simulink model "cosmic_ray_system_top"  (R2019a)
settings: Solver=VariableStepAuto  StartTime=0.0  StopTime=10.0  RelTol=1e-3
libraries: xbsIndex_r4 x3434, casper_library_misc x148, xps_library x3, casper_library_delays x1
(part 9 of 27)

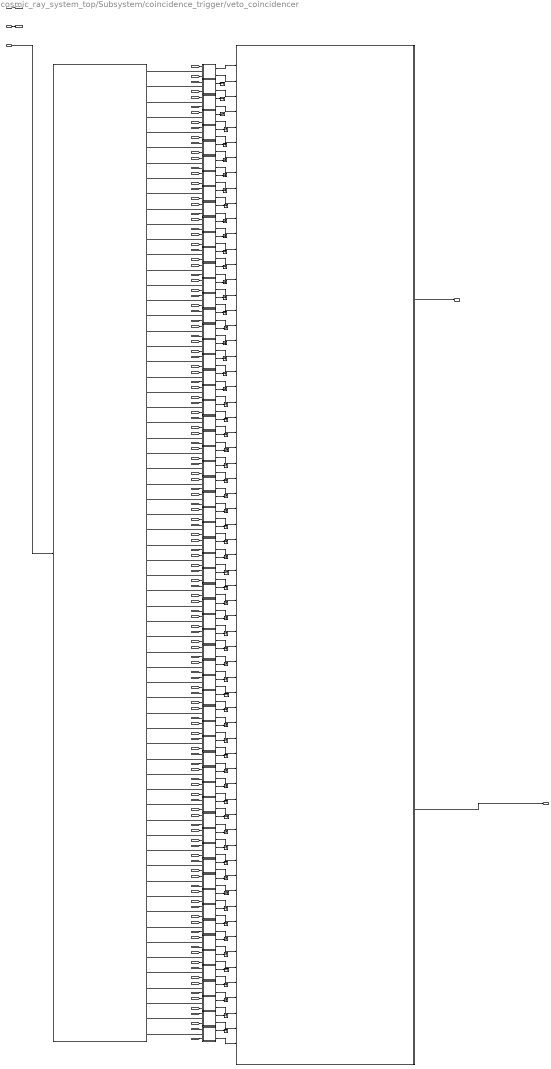
== system cosmic_ray_system_top/Subsystem/coincidence_trigger/veto_coincidencer ==
  window_length : Inport
  data_bus_in : Inport  Port=2
  sync_in : Inport  Port=3
  Terminator{,1..62} (63 alike) : Terminator
  adder_tree : Subsystem  AncestorBlock=casper_library_misc/adder_tree  mask(adder_tree){n_inputs=64, csp_latency=1, adder_imp=Fabric, first_stage_hdl=on, floating_point=off, dvalid_en=off, float_type=single, frac_width=0, exp_width=0}
      mask prompts: n_inputs "Number of Inputs"; csp_latency "Add Latency"; adder_imp "Adder implementation"; first_stage_hdl "Use behavioural HDL for first stage of adders"; floating_point "floating point"; float_type "float type"; frac_width "fraction length"; exp_width "exponent length"
      mask help:
      | Sums all inputs using a tree of adds and delays.
      |
      | Number of inputs: The number of inputs to the block to be summed
      | Add latency: The number of clock cycles to perform one addition (affects timing)..
      | Adder implementation: choice of fabric or DSP48E core, or behavioral HDL
      | Use behavioural HDL for first stage of adders: Causes the first stage of adders to be absorbed into DSP blocks if multipliers precede them (Virtex 5). Overrides Adder implementation
      mask init:
      | adder_tree_init(gcb, ...
      |     'n_inputs', n_inputs, ...
      |     'csp_latency', csp_latency, ...
      |     'adder_imp', adder_imp, ...
      |     'dvalid_en', dvalid_en, ...
      |     'floating_point', floating_point, ...
      |     'float_type', float_type, ...
      |     'exp_width', exp_width, ...
      |     'frac_width', frac_width, ...     
      |     'first_stage_hdl', first_stage_hdl);
      settings: AttributesFormatString=latency 6
      mask Help: eval('xlWeb(''http://casper.berkeley.edu/wiki/Adder_tree'')')
      mask TypeOptions adder_imp: Behavioral | Fabric | DSP48
      mask Callback floating_point:
      | onoff = get_param(gcb, 'floating_point');
      | if strcmp(onoff,'on')
      |     enable_fixpt = 'off'
      |     set_param_state(gcb, 'float_type', 'on')
      | 
      |     f_type = get_param(gcb, 'float_type')
      |     if strcmp(f_type,'custom')
      |         set_param_state(gcb, 'exp_width', 'on')
      |         set_param_state(gcb, 'frac_width', 'on')
      |     else
      |         set_param_state(gcb, 'exp_width', 'off')
      |         set_param_state(gcb, 'frac_width', 'off')
      |     end
      | 
      | 
      | else
      |     enable_fixpt = 'on'
      |     set_param_state(gcb, 'float_type', 'off')
      |     set_param_state(gcb, 'exp_width', 'off')
      |     set_param_state(gcb, 'frac_width', 'off')
      | end
      mask TypeOptions float_type: single | custom
      mask Callback float_type:
      | f_type = get_param(gcb, 'float_type')
      | if strcmp(f_type,'custom')
      |     set_param_state(gcb, 'exp_width', 'on')
      |     set_param_state(gcb, 'frac_width', 'on')
      | else
      |     set_param_state(gcb, 'exp_width', 'off')
      |     set_param_state(gcb, 'frac_width', 'off')
      | end
  bus_expand : Subsystem  AncestorBlock=casper_library_flow_control/bus_expand  mask(bus_expand){mode=divisions of equal size, outputNum=64, outputWidth=1, outputBinaryPt=0, outputArithmeticType=0, show_format=off, outputToWorkspace=off, variablePrefix=out, outputToModelAsWell=on}
      mask prompts: outputNum "Number of outputs:"; outputWidth "Output width:"; outputBinaryPt "Output binary point position:"; outputArithmeticType "Output arithmetic type (ufix=0, fix=1, bool=2):"; show_format "Print format string?"; outputToWorkspace "Output to workspace?"; variablePrefix "Variable name prefix:"; outputToModelAsWell "Output to model as well?"
      mask help:
      | Expands a 'bus' made using a bus_create or Xilinx
      | concat block.
      | The input will be divided into the specified number
      | of outputs with the specified arithmetic types.
      | Divisions are made from most significant bit.
      mask init: same as cosmic_ray_system_top/Subsystem/buffer_and_packetizer/bus_expand
      settings: AttributesFormatString=64 outputs
      mask TypeOptions mode: divisions of equal size | divisions of arbitrary size
      mask Callback mode: bus_expand_callback();
      mask Callback outputWidth: bus_expand_callback();
      mask Callback outputToWorkspace: bus_expand_callback();
  custom_pulse_extend_with_sync1 : Subsystem
  custom_pulse_extend_with_sync10 : Subsystem
  custom_pulse_extend_with_sync11 : Subsystem
  custom_pulse_extend_with_sync12 : Subsystem
  custom_pulse_extend_with_sync13 : Subsystem
  custom_pulse_extend_with_sync14 : Subsystem
  custom_pulse_extend_with_sync15 : Subsystem
  custom_pulse_extend_with_sync16 : Subsystem
  custom_pulse_extend_with_sync17 : Subsystem
  custom_pulse_extend_with_sync18 : Subsystem
  custom_pulse_extend_with_sync19 : Subsystem
  custom_pulse_extend_with_sync2 : Subsystem
  custom_pulse_extend_with_sync20 : Subsystem
  custom_pulse_extend_with_sync21 : Subsystem
  custom_pulse_extend_with_sync22 : Subsystem
  custom_pulse_extend_with_sync23 : Subsystem
  custom_pulse_extend_with_sync24 : Subsystem
  custom_pulse_extend_with_sync25 : Subsystem
  custom_pulse_extend_with_sync26 : Subsystem
  custom_pulse_extend_with_sync27 : Subsystem
  custom_pulse_extend_with_sync28 : Subsystem
  custom_pulse_extend_with_sync29 : Subsystem
  custom_pulse_extend_with_sync3 : Subsystem
  custom_pulse_extend_with_sync30 : Subsystem
  custom_pulse_extend_with_sync31 : Subsystem
  custom_pulse_extend_with_sync32 : Subsystem
  custom_pulse_extend_with_sync33 : Subsystem
  custom_pulse_extend_with_sync34 : Subsystem
  custom_pulse_extend_with_sync35 : Subsystem
  custom_pulse_extend_with_sync36 : Subsystem
  custom_pulse_extend_with_sync37 : Subsystem
  custom_pulse_extend_with_sync38 : Subsystem
  custom_pulse_extend_with_sync39 : Subsystem
  custom_pulse_extend_with_sync4 : Subsystem
  custom_pulse_extend_with_sync40 : Subsystem
  custom_pulse_extend_with_sync41 : Subsystem
  custom_pulse_extend_with_sync42 : Subsystem
  custom_pulse_extend_with_sync43 : Subsystem
  custom_pulse_extend_with_sync44 : Subsystem
  custom_pulse_extend_with_sync45 : Subsystem
  custom_pulse_extend_with_sync46 : Subsystem
  custom_pulse_extend_with_sync47 : Subsystem
  custom_pulse_extend_with_sync48 : Subsystem
  custom_pulse_extend_with_sync49 : Subsystem
  custom_pulse_extend_with_sync5 : Subsystem
  custom_pulse_extend_with_sync50 : Subsystem
  custom_pulse_extend_with_sync51 : Subsystem
  custom_pulse_extend_with_sync52 : Subsystem
  custom_pulse_extend_with_sync53 : Subsystem
  custom_pulse_extend_with_sync54 : Subsystem
  custom_pulse_extend_with_sync55 : Subsystem
  custom_pulse_extend_with_sync56 : Subsystem
  custom_pulse_extend_with_sync57 : Subsystem
  custom_pulse_extend_with_sync58 : Subsystem
  custom_pulse_extend_with_sync59 : Subsystem
  custom_pulse_extend_with_sync6 : Subsystem
  custom_pulse_extend_with_sync60 : Subsystem
  custom_pulse_extend_with_sync61 : Subsystem
  custom_pulse_extend_with_sync62 : Subsystem
  custom_pulse_extend_with_sync63 : Subsystem
  custom_pulse_extend_with_sync64 : Subsystem
  custom_pulse_extend_with_sync7 : Subsystem
  custom_pulse_extend_with_sync8 : Subsystem
  custom_pulse_extend_with_sync9 : Subsystem
  sync_out : Outport
  "out " : Outport  Port=2
  wires:
  custom_pulse_extend_with_sync2/1(sync_out) -> adder_tree/1(sync)
  adder_tree/1(sync_out) -> sync_out/1
  adder_tree/2(dout) -> "out "/1
  data_bus_in/1 -> bus_expand/1(bus_in)
  bus_expand/1(msb_out64) -> custom_pulse_extend_with_sync2/2("in ")
  window_length/1 -> [len]
  sync_in/1 -> [sync]
  [sync] -> custom_pulse_extend_with_sync2/1(sync_in)
  [len] -> custom_pulse_extend_with_sync2/3("pulse_length ")
  [len] -> custom_pulse_extend_with_sync1/3("pulse_length ")
  [sync] -> custom_pulse_extend_with_sync1/1(sync_in)
  bus_expand/2(out63) -> custom_pulse_extend_with_sync1/2("in ")
  bus_expand/4(out61) -> custom_pulse_extend_with_sync3/2("in ")
  [sync] -> custom_pulse_extend_with_sync3/1(sync_in)
  [len] -> custom_pulse_extend_with_sync3/3("pulse_length ")
  [len] -> custom_pulse_extend_with_sync4/3("pulse_length ")
  [sync] -> custom_pulse_extend_with_sync4/1(sync_in)
  bus_expand/3(out62) -> custom_pulse_extend_with_sync4/2("in ")
  bus_expand/7(out58) -> custom_pulse_extend_with_sync8/2("in ")
  [sync] -> custom_pulse_extend_with_sync8/1(sync_in)
  [len] -> custom_pulse_extend_with_sync8/3("pulse_length ")
  [len] -> custom_pulse_extend_with_sync7/3("pulse_length ")
  [sync] -> custom_pulse_extend_with_sync7/1(sync_in)
  bus_expand/8(out57) -> custom_pulse_extend_with_sync7/2("in ")
  bus_expand/6(out59) -> custom_pulse_extend_with_sync5/2("in ")
  [sync] -> custom_pulse_extend_with_sync5/1(sync_in)
  [len] -> custom_pulse_extend_with_sync5/3("pulse_length ")
  [len] -> custom_pulse_extend_with_sync6/3("pulse_length ")
  [sync] -> custom_pulse_extend_with_sync6/1(sync_in)
  bus_expand/5(out60) -> custom_pulse_extend_with_sync6/2("in ")
  bus_expand/12(out53) -> custom_pulse_extend_with_sync13/2("in ")
  [sync] -> custom_pulse_extend_with_sync13/1(sync_in)
  [len] -> custom_pulse_extend_with_sync13/3("pulse_length ")
  [len] -> custom_pulse_extend_with_sync12/3("pulse_length ")
  [sync] -> custom_pulse_extend_with_sync12/1(sync_in)
  bus_expand/13(out52) -> custom_pulse_extend_with_sync12/2("in ")
  bus_expand/15(out50) -> custom_pulse_extend_with_sync14/2("in ")
  [sync] -> custom_pulse_extend_with_sync14/1(sync_in)
  [len] -> custom_pulse_extend_with_sync14/3("pulse_length ")
  [len] -> custom_pulse_extend_with_sync15/3("pulse_length ")
  [sync] -> custom_pulse_extend_with_sync15/1(sync_in)
  bus_expand/14(out51) -> custom_pulse_extend_with_sync15/2("in ")
  bus_expand/10(out55) -> custom_pulse_extend_with_sync11/2("in ")
  [sync] -> custom_pulse_extend_with_sync11/1(sync_in)
  [len] -> custom_pulse_extend_with_sync11/3("pulse_length ")
  [len] -> custom_pulse_extend_with_sync10/3("pulse_length ")
  [sync] -> custom_pulse_extend_with_sync10/1(sync_in)
  bus_expand/11(out54) -> custom_pulse_extend_with_sync10/2("in ")
  bus_expand/9(out56) -> custom_pulse_extend_with_sync9/2("in ")
  [sync] -> custom_pulse_extend_with_sync9/1(sync_in)
  [len] -> custom_pulse_extend_with_sync9/3("pulse_length ")
  [len] -> custom_pulse_extend_with_sync30/3("pulse_length ")
  [sync] -> custom_pulse_extend_with_sync30/1(sync_in)
  bus_expand/24(out41) -> custom_pulse_extend_with_sync30/2("in ")
  bus_expand/26(out39) -> custom_pulse_extend_with_sync17/2("in ")
  [sync] -> custom_pulse_extend_with_sync17/1(sync_in)
  [len] -> custom_pulse_extend_with_sync17/3("pulse_length ")
  [len] -> custom_pulse_extend_with_sync18/3("pulse_length ")
  [sync] -> custom_pulse_extend_with_sync18/1(sync_in)
  bus_expand/25(out40) -> custom_pulse_extend_with_sync18/2("in ")
  bus_expand/29(out36) -> custom_pulse_extend_with_sync22/2("in ")
  [sync] -> custom_pulse_extend_with_sync22/1(sync_in)
  [len] -> custom_pulse_extend_with_sync22/3("pulse_length ")
  [len] -> custom_pulse_extend_with_sync21/3("pulse_length ")
  [sync] -> custom_pulse_extend_with_sync21/1(sync_in)
  bus_expand/30(out35) -> custom_pulse_extend_with_sync21/2("in ")
  bus_expand/28(out37) -> custom_pulse_extend_with_sync19/2("in ")
  [sync] -> custom_pulse_extend_with_sync19/1(sync_in)
  [len] -> custom_pulse_extend_with_sync19/3("pulse_length ")
  [len] -> custom_pulse_extend_with_sync20/3("pulse_length ")
  [sync] -> custom_pulse_extend_with_sync20/1(sync_in)
  bus_expand/27(out38) -> custom_pulse_extend_with_sync20/2("in ")
  bus_expand/20(out45) -> custom_pulse_extend_with_sync27/2("in ")
  [sync] -> custom_pulse_extend_with_sync27/1(sync_in)
  [len] -> custom_pulse_extend_with_sync27/3("pulse_length ")
  [len] -> custom_pulse_extend_with_sync26/3("pulse_length ")
  [sync] -> custom_pulse_extend_with_sync26/1(sync_in)
  bus_expand/21(out44) -> custom_pulse_extend_with_sync26/2("in ")
  bus_expand/23(out42) -> custom_pulse_extend_with_sync28/2("in ")
  [sync] -> custom_pulse_extend_with_sync28/1(sync_in)
  [len] -> custom_pulse_extend_with_sync28/3("pulse_length ")
  [len] -> custom_pulse_extend_with_sync29/3("pulse_length ")
  [sync] -> custom_pulse_extend_with_sync29/1(sync_in)
  bus_expand/22(out43) -> custom_pulse_extend_with_sync29/2("in ")
  bus_expand/18(out47) -> custom_pulse_extend_with_sync25/2("in ")
  [sync] -> custom_pulse_extend_with_sync25/1(sync_in)
  [len] -> custom_pulse_extend_with_sync25/3("pulse_length ")
  [len] -> custom_pulse_extend_with_sync24/3("pulse_length ")
  [sync] -> custom_pulse_extend_with_sync24/1(sync_in)
  bus_expand/19(out46) -> custom_pulse_extend_with_sync24/2("in ")
  bus_expand/17(out48) -> custom_pulse_extend_with_sync16/2("in ")
  [sync] -> custom_pulse_extend_with_sync16/1(sync_in)
  [len] -> custom_pulse_extend_with_sync16/3("pulse_length ")
  [len] -> custom_pulse_extend_with_sync23/3("pulse_length ")
  [sync] -> custom_pulse_extend_with_sync23/1(sync_in)
  bus_expand/16(out49) -> custom_pulse_extend_with_sync23/2("in ")
  bus_expand/46(out19) -> custom_pulse_extend_with_sync46/2("in ")
  [sync] -> custom_pulse_extend_with_sync46/1(sync_in)
  [len] -> custom_pulse_extend_with_sync46/3("pulse_length ")
  [len] -> custom_pulse_extend_with_sync38/3("pulse_length ")
  [sync] -> custom_pulse_extend_with_sync38/1(sync_in)
  bus_expand/47(out18) -> custom_pulse_extend_with_sync38/2("in ")
  bus_expand/49(out16) -> custom_pulse_extend_with_sync47/2("in ")
  [sync] -> custom_pulse_extend_with_sync47/1(sync_in)
  [len] -> custom_pulse_extend_with_sync47/3("pulse_length ")
  [len] -> custom_pulse_extend_with_sync48/3("pulse_length ")
  [sync] -> custom_pulse_extend_with_sync48/1(sync_in)
  bus_expand/48(out17) -> custom_pulse_extend_with_sync48/2("in ")
  bus_expand/52(out13) -> custom_pulse_extend_with_sync52/2("in ")
  [sync] -> custom_pulse_extend_with_sync52/1(sync_in)
  [len] -> custom_pulse_extend_with_sync52/3("pulse_length ")
  [len] -> custom_pulse_extend_with_sync51/3("pulse_length ")
  [sync] -> custom_pulse_extend_with_sync51/1(sync_in)
  bus_expand/53(out12) -> custom_pulse_extend_with_sync51/2("in ")
  bus_expand/51(out14) -> custom_pulse_extend_with_sync49/2("in ")
  [sync] -> custom_pulse_extend_with_sync49/1(sync_in)
  [len] -> custom_pulse_extend_with_sync49/3("pulse_length ")
  [len] -> custom_pulse_extend_with_sync50/3("pulse_length ")
  [sync] -> custom_pulse_extend_with_sync50/1(sync_in)
  bus_expand/50(out15) -> custom_pulse_extend_with_sync50/2("in ")
  bus_expand/57(out8) -> custom_pulse_extend_with_sync43/2("in ")
  [sync] -> custom_pulse_extend_with_sync43/1(sync_in)
  [len] -> custom_pulse_extend_with_sync43/3("pulse_length ")
  [len] -> custom_pulse_extend_with_sync41/3("pulse_length ")
  [sync] -> custom_pulse_extend_with_sync41/1(sync_in)
  bus_expand/58(out7) -> custom_pulse_extend_with_sync41/2("in ")
  bus_expand/60(out5) -> custom_pulse_extend_with_sync44/2("in ")
  [sync] -> custom_pulse_extend_with_sync44/1(sync_in)
  [len] -> custom_pulse_extend_with_sync44/3("pulse_length ")
  [len] -> custom_pulse_extend_with_sync45/3("pulse_length ")
  [sync] -> custom_pulse_extend_with_sync45/1(sync_in)
  bus_expand/59(out6) -> custom_pulse_extend_with_sync45/2("in ")
  bus_expand/55(out10) -> custom_pulse_extend_with_sync40/2("in ")
  [sync] -> custom_pulse_extend_with_sync40/1(sync_in)
  [len] -> custom_pulse_extend_with_sync40/3("pulse_length ")
  [len] -> custom_pulse_extend_with_sync39/3("pulse_length ")
  [sync] -> custom_pulse_extend_with_sync39/1(sync_in)
  bus_expand/56(out9) -> custom_pulse_extend_with_sync39/2("in ")
  bus_expand/54(out11) -> custom_pulse_extend_with_sync54/2("in ")
  [sync] -> custom_pulse_extend_with_sync54/1(sync_in)
  [len] -> custom_pulse_extend_with_sync54/3("pulse_length ")
  [len] -> custom_pulse_extend_with_sync60/3("pulse_length ")
  [sync] -> custom_pulse_extend_with_sync60/1(sync_in)
  bus_expand/39(out26) -> custom_pulse_extend_with_sync60/2("in ")
  bus_expand/41(out24) -> custom_pulse_extend_with_sync32/2("in ")
  [sync] -> custom_pulse_extend_with_sync32/1(sync_in)
  [len] -> custom_pulse_extend_with_sync32/3("pulse_length ")
  [len] -> custom_pulse_extend_with_sync33/3("pulse_length ")
  [sync] -> custom_pulse_extend_with_sync33/1(sync_in)
  bus_expand/40(out25) -> custom_pulse_extend_with_sync33/2("in ")
  bus_expand/44(out21) -> custom_pulse_extend_with_sync37/2("in ")
  [sync] -> custom_pulse_extend_with_sync37/1(sync_in)
  [len] -> custom_pulse_extend_with_sync37/3("pulse_length ")
  [len] -> custom_pulse_extend_with_sync36/3("pulse_length ")
  [sync] -> custom_pulse_extend_with_sync36/1(sync_in)
  bus_expand/45(out20) -> custom_pulse_extend_with_sync36/2("in ")
  bus_expand/43(out22) -> custom_pulse_extend_with_sync34/2("in ")
  [sync] -> custom_pulse_extend_with_sync34/1(sync_in)
  [len] -> custom_pulse_extend_with_sync34/3("pulse_length ")
  [len] -> custom_pulse_extend_with_sync35/3("pulse_length ")
  [sync] -> custom_pulse_extend_with_sync35/1(sync_in)
  bus_expand/42(out23) -> custom_pulse_extend_with_sync35/2("in ")
  bus_expand/35(out30) -> custom_pulse_extend_with_sync57/2("in ")
  [sync] -> custom_pulse_extend_with_sync57/1(sync_in)
  [len] -> custom_pulse_extend_with_sync57/3("pulse_length ")
  [len] -> custom_pulse_extend_with_sync56/3("pulse_length ")
  [sync] -> custom_pulse_extend_with_sync56/1(sync_in)
  bus_expand/36(out29) -> custom_pulse_extend_with_sync56/2("in ")
  bus_expand/38(out27) -> custom_pulse_extend_with_sync58/2("in ")
  [sync] -> custom_pulse_extend_with_sync58/1(sync_in)
  [len] -> custom_pulse_extend_with_sync58/3("pulse_length ")
  [len] -> custom_pulse_extend_with_sync59/3("pulse_length ")
  [sync] -> custom_pulse_extend_with_sync59/1(sync_in)
  bus_expand/37(out28) -> custom_pulse_extend_with_sync59/2("in ")
  bus_expand/33(out32) -> custom_pulse_extend_with_sync55/2("in ")
  [sync] -> custom_pulse_extend_with_sync55/1(sync_in)
  [len] -> custom_pulse_extend_with_sync55/3("pulse_length ")
  [len] -> custom_pulse_extend_with_sync53/3("pulse_length ")
  [sync] -> custom_pulse_extend_with_sync53/1(sync_in)
  bus_expand/34(out31) -> custom_pulse_extend_with_sync53/2("in ")
  bus_expand/32(out33) -> custom_pulse_extend_with_sync31/2("in ")
  [sync] -> custom_pulse_extend_with_sync31/1(sync_in)
  [len] -> custom_pulse_extend_with_sync31/3("pulse_length ")
  [len] -> custom_pulse_extend_with_sync42/3("pulse_length ")
  [sync] -> custom_pulse_extend_with_sync42/1(sync_in)
  bus_expand/31(out34) -> custom_pulse_extend_with_sync42/2("in ")
  bus_expand/63(out2) -> custom_pulse_extend_with_sync64/2("in ")
  [sync] -> custom_pulse_extend_with_sync64/1(sync_in)
  [len] -> custom_pulse_extend_with_sync64/3("pulse_length ")
  [len] -> custom_pulse_extend_with_sync63/3("pulse_length ")
  [sync] -> custom_pulse_extend_with_sync63/1(sync_in)
  bus_expand/64(lsb_out1) -> custom_pulse_extend_with_sync63/2("in ")
  bus_expand/62(out3) -> custom_pulse_extend_with_sync61/2("in ")
  [sync] -> custom_pulse_extend_with_sync61/1(sync_in)
  [len] -> custom_pulse_extend_with_sync61/3("pulse_length ")
  [len] -> custom_pulse_extend_with_sync62/3("pulse_length ")
  [sync] -> custom_pulse_extend_with_sync62/1(sync_in)
  bus_expand/61(out4) -> custom_pulse_extend_with_sync62/2("in ")
  custom_pulse_extend_with_sync1/1(sync_out) -> Terminator/1
  custom_pulse_extend_with_sync4/1(sync_out) -> Terminator1/1
  custom_pulse_extend_with_sync3/1(sync_out) -> Terminator2/1
  custom_pulse_extend_with_sync6/1(sync_out) -> Terminator3/1
  custom_pulse_extend_with_sync5/1(sync_out) -> Terminator4/1
  custom_pulse_extend_with_sync8/1(sync_out) -> Terminator5/1
  custom_pulse_extend_with_sync7/1(sync_out) -> Terminator6/1
  custom_pulse_extend_with_sync9/1(sync_out) -> Terminator7/1
  custom_pulse_extend_with_sync15/1(sync_out) -> Terminator12/1
  custom_pulse_extend_with_sync12/1(sync_out) -> Terminator11/1
  custom_pulse_extend_with_sync13/1(sync_out) -> Terminator10/1
  custom_pulse_extend_with_sync10/1(sync_out) -> Terminator9/1
  custom_pulse_extend_with_sync11/1(sync_out) -> Terminator8/1
  custom_pulse_extend_with_sync25/1(sync_out) -> Terminator19/1
  custom_pulse_extend_with_sync24/1(sync_out) -> Terminator20/1
  custom_pulse_extend_with_sync27/1(sync_out) -> Terminator13/1
  custom_pulse_extend_with_sync26/1(sync_out) -> Terminator14/1
  custom_pulse_extend_with_sync29/1(sync_out) -> Terminator15/1
  custom_pulse_extend_with_sync16/1(sync_out) -> Terminator18/1
  custom_pulse_extend_with_sync23/1(sync_out) -> Terminator17/1
  custom_pulse_extend_with_sync14/1(sync_out) -> Terminator16/1
  custom_pulse_extend_with_sync28/1(sync_out) -> Terminator24/1
  custom_pulse_extend_with_sync30/1(sync_out) -> Terminator25/1
  custom_pulse_extend_with_sync18/1(sync_out) -> Terminator26/1
  custom_pulse_extend_with_sync21/1(sync_out) -> Terminator23/1
  custom_pulse_extend_with_sync22/1(sync_out) -> Terminator22/1
  custom_pulse_extend_with_sync19/1(sync_out) -> Terminator21/1
  custom_pulse_extend_with_sync20/1(sync_out) -> Terminator28/1
  custom_pulse_extend_with_sync17/1(sync_out) -> Terminator27/1
  custom_pulse_extend_with_sync53/1(sync_out) -> Terminator35/1
  custom_pulse_extend_with_sync57/1(sync_out) -> Terminator36/1
  custom_pulse_extend_with_sync56/1(sync_out) -> Terminator29/1
  custom_pulse_extend_with_sync59/1(sync_out) -> Terminator30/1
  custom_pulse_extend_with_sync58/1(sync_out) -> Terminator31/1
  custom_pulse_extend_with_sync55/1(sync_out) -> Terminator34/1
  custom_pulse_extend_with_sync31/1(sync_out) -> Terminator33/1
  custom_pulse_extend_with_sync42/1(sync_out) -> Terminator32/1
  custom_pulse_extend_with_sync38/1(sync_out) -> Terminator48/1
  custom_pulse_extend_with_sync48/1(sync_out) -> Terminator49/1
  custom_pulse_extend_with_sync47/1(sync_out) -> Terminator50/1
  custom_pulse_extend_with_sync54/1(sync_out) -> Terminator47/1
  custom_pulse_extend_with_sync51/1(sync_out) -> Terminator46/1
  custom_pulse_extend_with_sync52/1(sync_out) -> Terminator45/1
  custom_pulse_extend_with_sync49/1(sync_out) -> Terminator52/1
  custom_pulse_extend_with_sync50/1(sync_out) -> Terminator51/1
  custom_pulse_extend_with_sync35/1(sync_out) -> Terminator43/1
  custom_pulse_extend_with_sync34/1(sync_out) -> Terminator44/1
  custom_pulse_extend_with_sync37/1(sync_out) -> Terminator37/1
  custom_pulse_extend_with_sync36/1(sync_out) -> Terminator38/1
  custom_pulse_extend_with_sync46/1(sync_out) -> Terminator39/1
  custom_pulse_extend_with_sync32/1(sync_out) -> Terminator42/1
  custom_pulse_extend_with_sync33/1(sync_out) -> Terminator41/1
  custom_pulse_extend_with_sync60/1(sync_out) -> Terminator40/1
  custom_pulse_extend_with_sync40/1(sync_out) -> Terminator56/1
  custom_pulse_extend_with_sync39/1(sync_out) -> Terminator57/1
  custom_pulse_extend_with_sync43/1(sync_out) -> Terminator53/1
  custom_pulse_extend_with_sync41/1(sync_out) -> Terminator54/1
  custom_pulse_extend_with_sync45/1(sync_out) -> Terminator55/1
  custom_pulse_extend_with_sync63/1(sync_out) -> Terminator60/1
  custom_pulse_extend_with_sync64/1(sync_out) -> Terminator59/1
  custom_pulse_extend_with_sync61/1(sync_out) -> Terminator58/1
  custom_pulse_extend_with_sync62/1(sync_out) -> Terminator62/1
  custom_pulse_extend_with_sync44/1(sync_out) -> Terminator61/1
  custom_pulse_extend_with_sync2/2("out ") -> adder_tree/2(din1)
  custom_pulse_extend_with_sync1/2("out ") -> adder_tree/3(din2)
  custom_pulse_extend_with_sync4/2("out ") -> adder_tree/4(din3)
  custom_pulse_extend_with_sync3/2("out ") -> adder_tree/5(din4)
  custom_pulse_extend_with_sync6/2("out ") -> adder_tree/6(din5)
  custom_pulse_extend_with_sync5/2("out ") -> adder_tree/7(din6)
  custom_pulse_extend_with_sync8/2("out ") -> adder_tree/8(din7)
  custom_pulse_extend_with_sync7/2("out ") -> adder_tree/9(din8)
  custom_pulse_extend_with_sync9/2("out ") -> adder_tree/10(din9)
  custom_pulse_extend_with_sync11/2("out ") -> adder_tree/11(din10)
  custom_pulse_extend_with_sync10/2("out ") -> adder_tree/12(din11)
  custom_pulse_extend_with_sync13/2("out ") -> adder_tree/13(din12)
  custom_pulse_extend_with_sync12/2("out ") -> adder_tree/14(din13)
  custom_pulse_extend_with_sync15/2("out ") -> adder_tree/15(din14)
  custom_pulse_extend_with_sync14/2("out ") -> adder_tree/16(din15)
  custom_pulse_extend_with_sync23/2("out ") -> adder_tree/17(din16)
  custom_pulse_extend_with_sync16/2("out ") -> adder_tree/18(din17)
  custom_pulse_extend_with_sync25/2("out ") -> adder_tree/19(din18)
  custom_pulse_extend_with_sync24/2("out ") -> adder_tree/20(din19)
  custom_pulse_extend_with_sync27/2("out ") -> adder_tree/21(din20)
  custom_pulse_extend_with_sync26/2("out ") -> adder_tree/22(din21)
  custom_pulse_extend_with_sync29/2("out ") -> adder_tree/23(din22)
  custom_pulse_extend_with_sync28/2("out ") -> adder_tree/24(din23)
  custom_pulse_extend_with_sync30/2("out ") -> adder_tree/25(din24)
  custom_pulse_extend_with_sync18/2("out ") -> adder_tree/26(din25)
  custom_pulse_extend_with_sync17/2("out ") -> adder_tree/27(din26)
  custom_pulse_extend_with_sync20/2("out ") -> adder_tree/28(din27)
  custom_pulse_extend_with_sync19/2("out ") -> adder_tree/29(din28)
  custom_pulse_extend_with_sync22/2("out ") -> adder_tree/30(din29)
  custom_pulse_extend_with_sync21/2("out ") -> adder_tree/31(din30)
  custom_pulse_extend_with_sync42/2("out ") -> adder_tree/32(din31)
  custom_pulse_extend_with_sync31/2("out ") -> adder_tree/33(din32)
  custom_pulse_extend_with_sync55/2("out ") -> adder_tree/34(din33)
  custom_pulse_extend_with_sync53/2("out ") -> adder_tree/35(din34)
  custom_pulse_extend_with_sync57/2("out ") -> adder_tree/36(din35)
  custom_pulse_extend_with_sync56/2("out ") -> adder_tree/37(din36)
  custom_pulse_extend_with_sync59/2("out ") -> adder_tree/38(din37)
  custom_pulse_extend_with_sync58/2("out ") -> adder_tree/39(din38)
  custom_pulse_extend_with_sync60/2("out ") -> adder_tree/40(din39)
  custom_pulse_extend_with_sync33/2("out ") -> adder_tree/41(din40)
  custom_pulse_extend_with_sync32/2("out ") -> adder_tree/42(din41)
  custom_pulse_extend_with_sync35/2("out ") -> adder_tree/43(din42)
  custom_pulse_extend_with_sync34/2("out ") -> adder_tree/44(din43)
  custom_pulse_extend_with_sync37/2("out ") -> adder_tree/45(din44)
  custom_pulse_extend_with_sync36/2("out ") -> adder_tree/46(din45)
  custom_pulse_extend_with_sync46/2("out ") -> adder_tree/47(din46)
  custom_pulse_extend_with_sync38/2("out ") -> adder_tree/48(din47)
  custom_pulse_extend_with_sync48/2("out ") -> adder_tree/49(din48)
  custom_pulse_extend_with_sync47/2("out ") -> adder_tree/50(din49)
  custom_pulse_extend_with_sync50/2("out ") -> adder_tree/51(din50)
  custom_pulse_extend_with_sync49/2("out ") -> adder_tree/52(din51)
  custom_pulse_extend_with_sync52/2("out ") -> adder_tree/53(din52)
  custom_pulse_extend_with_sync51/2("out ") -> adder_tree/54(din53)
  custom_pulse_extend_with_sync54/2("out ") -> adder_tree/55(din54)
  custom_pulse_extend_with_sync40/2("out ") -> adder_tree/56(din55)
  custom_pulse_extend_with_sync39/2("out ") -> adder_tree/57(din56)
  custom_pulse_extend_with_sync43/2("out ") -> adder_tree/58(din57)
  custom_pulse_extend_with_sync41/2("out ") -> adder_tree/59(din58)
  custom_pulse_extend_with_sync45/2("out ") -> adder_tree/60(din59)
  custom_pulse_extend_with_sync44/2("out ") -> adder_tree/61(din60)
  custom_pulse_extend_with_sync62/2("out ") -> adder_tree/62(din61)
  custom_pulse_extend_with_sync61/2("out ") -> adder_tree/63(din62)
  custom_pulse_extend_with_sync64/2("out ") -> adder_tree/64(din63)
  custom_pulse_extend_with_sync63/2("out ") -> adder_tree/65(din64)
